simulink model "ramos_dynamic_bilateral_telo_sim"  (R2019a)
settings: Solver=VariableStepAuto  StartTime=0.0  StopTime=10.0  RelTol=1e-3
values from neighbouring files (symbols this model uses):
  D = ?    [lqr_controllers.m]
  K = 0    [Eqs_of_motion_from_lagrangian_bottom_up_FINAL.m]    (also in lqr_controllers.m = cell(1,52))
undefined symbols (not defined in the file or in its folder): A_r_, B_r, C_1, C_2, C_3, C_4, q_ref
settings Model: Creator=purusho2  LastModifiedBy=purusho2

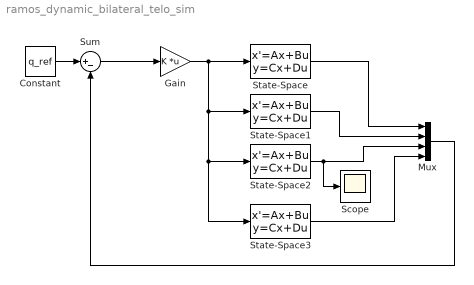
== system ramos_dynamic_bilateral_telo_sim ==
  Constant : Constant  Value=q_ref
  Gain : Gain  Gain=K  Multiplication=Matrix(K*u) (u vector)
  Mux : Mux
  Scope : Scope
  State-Space : StateSpace  A=A_r_  B=B_r  C=C_1  D=D  InitialCondition=0
  State-Space1 : StateSpace  A=A_r_  B=B_r  C=C_2  D=D  InitialCondition=0
  State-Space2 : StateSpace  A=A_r_  B=B_r  C=C_3  D=D  InitialCondition=0
  State-Space3 : StateSpace  A=A_r_  B=B_r  C=C_4  D=D  InitialCondition=0
  Sum : Sum  Inputs=|+-
  wires:
  Constant/1 -> Sum/1
  State-Space/1 -> Mux/1
  State-Space1/1 -> Mux/2
  State-Space2/1 -> Scope/1, Mux/3
  State-Space3/1 -> Mux/4
  Mux/1 -> Sum/2
  Sum/1 -> Gain/1
  Gain/1 -> State-Space3/1, State-Space2/1, State-Space1/1, State-Space/1
